simulink model "Four_Short_Circuit_test_on_3ph_Transformer"  (R2024a)
settings: Solver=ode23tb  StartTime=0.0  StopTime=0.2  MaxStep=1e-4  RelTol=1e-3
libraries: spsACVoltageSourceLib x3, spsRMSLib x2, spsGroundLib x1, spsPower3phInstantaneousLib x1, spsThreePhaseTransformerTwoWindingsLib x1, spsThreePhaseVIMeasurementLib x1, spspowerguiLib x1
settings Model: Creator=91889  LastModifiedBy=91889

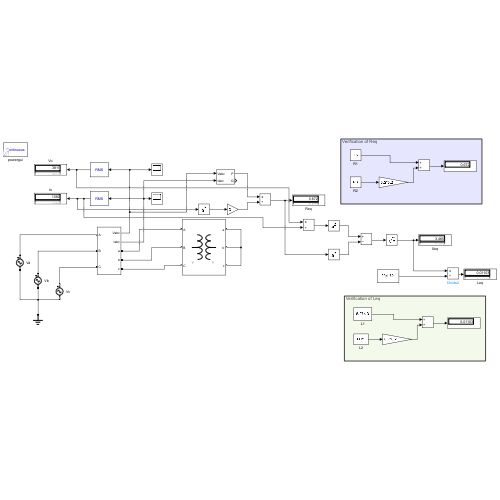
[thumbnail: Simulink's stored preview of the top-level diagram]
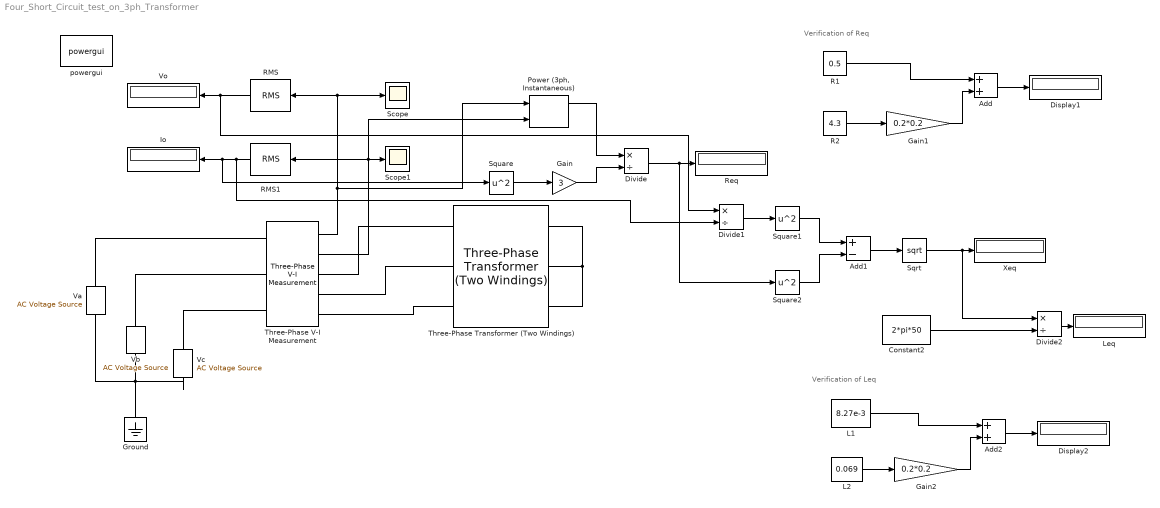
== system Four_Short_Circuit_test_on_3ph_Transformer ==
  note: Verification of Req
  note: Verification of Leq
  Add : Sum
  Add1 : Sum  Inputs=+-
  Add2 : Sum
  Constant2 : Constant  Value=2*pi*50
  Display1 : Display
  Display2 : Display
  Divide : Product  Inputs=*/
  Divide1 : Product  Inputs=*/
  Divide2 : Product  Inputs=*/
  Gain : Gain  Gain=3
  Gain1 : Gain  Gain=0.2*0.2
  Gain2 : Gain  Gain=0.2*0.2
  Ground : spsGroundLib/Ground  LConnTagsString=a
  Io : Display
  L1 : Constant  Value=8.27e-3
  L2 : Constant  Value=0.069
  Leq : Display
  "Power (3ph, Instantaneous)" : spsPower3phInstantaneousLib/Power (3ph, Instantaneous)
  R1 : Constant  Value=0.5
  R2 : Constant  Value=4.3
  RMS : spsRMSLib/RMS  TrueRMS=off  Freq=50  RMSInit=0  Ts=0
  RMS1 : spsRMSLib/RMS  TrueRMS=off  Freq=50  RMSInit=0  Ts=0
  Req : Display
  Scope : Scope
  Scope1 : Scope
  Sqrt : Sqrt
  Square : Math  Operator=square
  Square1 : Math  Operator=square
  Square2 : Math  Operator=square
  Three-Phase Transformer (Two Windings) : spsThreePhaseTransformerTwoWindingsLib/Three-Phase Transformer (Two Windings)  Winding1Connection=Y  Winding2Connection=Y  CoreType=Three single-phase transformers  SetSaturation=off  Hysteresis=off  DataFile='hysteresis'  SetInitialFlux=off  Measurements=None  UNITS=SI  NominalPower=[ 2000e3 , 50 ]  Winding1=[6.6e3 0.5 8.27e-3]  Winding2=[33e3 4.3 0.069]  Rm=10000  Lm=500  L0=0.5  Saturation=[0 0;0.59382 20.584;247.42 26.073]  InitialFluxes=[13.723 -13.723 12.007]  BreakLoop=off  DiscreteSolver=Trapezoidal iterative  DataType=on  TransfoNumber=1
  Three-Phase V-I Measurement : spsThreePhaseVIMeasurementLib/Three-Phase V-I Measurement  VoltageMeasurement=phase-to-ground  SetLabelV=off  LabelV=Vabc  Vpu=off  VpuLL=off  CurrentMeasurement=yes  SetLabelI=off  LabelI=Iabc  Ipu=off  Pbase=100e6  Vbase=500e3  OutputType=Complex  PhasorSimulation=off  PSBequivalent=0
  Va : spsACVoltageSourceLib/AC Voltage Source  Amplitude=6.6*1000*sqrt(2)/sqrt(3)  Phase=0  Frequency=50  SampleTime=0  Measurements=None  BusType=swing  Pref=10e3  Qref=0  Qmin=-inf  Qmax=+inf
  Vb : spsACVoltageSourceLib/AC Voltage Source  Amplitude=6.6*1000*sqrt(2)/sqrt(3)  Phase=-120  Frequency=50  SampleTime=0  Measurements=None  BusType=swing  Pref=10e3  Qref=0  Qmin=-inf  Qmax=+inf
  Vc : spsACVoltageSourceLib/AC Voltage Source  Amplitude=6.6*1000*sqrt(2)/sqrt(3)  Phase=120  Frequency=50  SampleTime=0  Measurements=None  BusType=swing  Pref=10e3  Qref=0  Qmin=-inf  Qmax=+inf
  Vo : Display
  Xeq : Display
  powergui : spspowerguiLib/powergui  Priority=1  SimulationMode=Continuous  SampleTime=50e-6  frequency=60  Iterations=50  frequencyindice=50  Pbase=100e6  ErrMax=1e-4  UnitsV=kV  UnitsW=MW  buscounter=0  FunctionMessages=off  echomessages=off  EnableUseOfTLC=off  CurrentSourceSwitches=off  DisableSnubberDevices=off  DisableRonSwitches=off  DisableVfSwitches=off  DisplayEquations=off  AutomaticDiscreteSolvers=off  SolverType=Tustin/Backward Euler (TBE)  Interpol=off  ExternalGateDelay=off  methode=off  Ts=100  x0status=blocks  SPID=off  SwTol=0  HookPort=off  NonlinearTolerance=1e-4  nMaxIteration=100  ContinueOnMaxIteration=off  RestoreLinks=warning  ResistiveCurrentMeasurement=off  Frange=[0:2:500]  Ylog=off  Xlog=on  ShowGrid=off  save=off  variable=ZData  structure=0  ZoomFFT=off  StartTime=0.0  cycles=1  DisplayStyle=1  fundamental=60  FreqAxis=off  MaxFrequency=1000  frequencyindicesteady=1  RmsSteady=1  display=off
  wires:
  Three-Phase V-I Measurement/1 -> "Power (3ph, Instantaneous)"/1, Scope/1, RMS/1
  Three-Phase V-I Measurement/2 -> "Power (3ph, Instantaneous)"/2, Scope1/1, RMS1/1
  RMS/1 -> Divide1/1, Vo/1
  RMS1/1 -> Square/1, Io/1, Divide1/2
  "Power (3ph, Instantaneous)"/1 -> Divide/1
  Square/1 -> Gain/1
  Gain/1 -> Divide/2
  Divide/1 -> Square2/1, Req/1
  R2/1 -> Gain1/1
  R1/1 -> Add/1
  Gain1/1 -> Add/2
  Add/1 -> Display1/1
  Divide1/1 -> Square1/1
  Square1/1 -> Add1/1
  Square2/1 -> Add1/2
  Add1/1 -> Sqrt/1
  Sqrt/1 -> Divide2/1, Xeq/1
  Constant2/1 -> Divide2/2
  Divide2/1 -> Leq/1
  Add2/1 -> Display2/1
  Gain2/1 -> Add2/2
  L1/1 -> Add2/1
  L2/1 -> Gain2/1
  connections:
  Va/LConn1 -- Vc/LConn1 -- Ground/LConn1 -- Vb/LConn1
  Three-Phase V-I Measurement/RConn3 -- Three-Phase Transformer (Two Windings)/LConn3
  Three-Phase V-I Measurement/LConn2 -- Vb/RConn1
  Va/RConn1 -- Three-Phase V-I Measurement/LConn1
  Three-Phase V-I Measurement/RConn1 -- Three-Phase Transformer (Two Windings)/LConn1
  Three-Phase V-I Measurement/RConn2 -- Three-Phase Transformer (Two Windings)/LConn2
  Vc/RConn1 -- Three-Phase V-I Measurement/LConn3
  Three-Phase Transformer (Two Windings)/RConn1 -- Three-Phase Transformer (Two Windings)/RConn2 -- Three-Phase Transformer (Two Windings)/RConn3
